simulink model "simulacionrobusto"  (R2024a)
settings: Solver=FixedStepAuto  StartTime=0.0  StopTime=3  FixedStep=0.000001  RelTol=1e-3
model workspace (MAT data in the model file):
  tau = Simulink.Parameter
  tau.Complexity = 'real'
  tau.Dimensions = [0 0]
  tau.DataType = 'auto'
values from neighbouring files (symbols this model uses):
  C = 2610*10^-6    (= 0.00261)    [SITLparameters.m]
  delta1 = 0.022    [SITLparameters.m]
  delta2 = 0.012    [SITLparameters.m]
  E = 12    [SITLparameters.m]
  k1 = 10000    [SITLparameters.m]
  k2 = 280    [SITLparameters.m]
  k3 = 10    [SITLparameters.m]
  kl = 1    [SITLparameters.m]
  kp = 0.0019    [SITLparameters.m]
  kp1 = 0.0019    [SITLparameters.m]
  kp2 = 0.1    [SITLparameters.m]
  kp3 = 0.1    [SITLparameters.m]
  kr1 = 0    [SITLparameters.m]
  kr2 = 0    [SITLparameters.m]
  L = 2010*10^-6    (= 0.00201)    [SITLparameters.m]
  L1 = 0.91    [SITLparameters.m]
  M = 1    [SITLparameters.m]
  R = 25    [SITLparameters.m]
  vd = -8    [SITLparameters.m]
libraries: simulink x6, spsDCVoltageSourceLib x2, spsSawtoothGeneratorLib x2, spsSeriesRLCBranchLib x2, spsCurrentMeasurementLib x1, spsDiodeLib x1, spsMosfetLib x1, slpidlib x1, spsVariableResistorLib x1, spsVoltageMeasurementLib x1, spspowerguiLib x1
settings Model: Creator=LAPONE  LastModifiedBy=rodol
settings SolverCC: ZeroCrossAlgorithm=Adaptive
settings DebuggingCC: IgnoredZcDiagnostic=none  UnconnectedInputMsg=warning  UnconnectedOutputMsg=warning  UnconnectedLineMsg=warning
settings ModelReferenceCC: EnableRefExpFcnMdlSchedulingChecks=on
settings RTWCC: GPUComputeCapability=3.5  DLArmComputeVersion=19.05

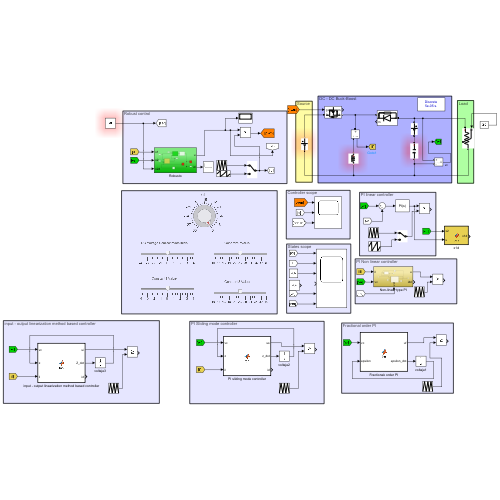
[thumbnail: Simulink's stored preview of the top-level diagram]
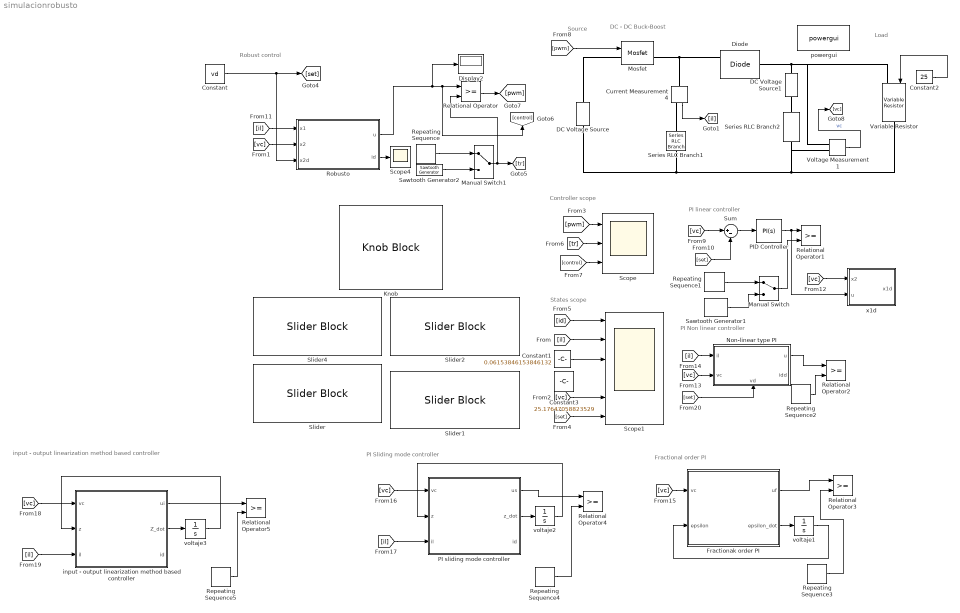
== system simulacionrobusto ==
  note: input - output linearization method based controller
  note: PI Sliding mode controller
  note: Controller scope
  note: States scope
  note: DC - DC Buck-Boost
  note: Robust control
  note: PI linear controller
  note: Load
  note: Source
  note: PI Non linear controller
  note: Fractional order PI
  Constant : Constant  Value=vd
  Constant1 : Constant  Value=0.06153846153846132
  Constant2 : Constant  Value=25
  Constant3 : Constant  Value=25.17647058823529
  Current Measurement4 : spsCurrentMeasurementLib/Current Measurement  PhasorSimulation=off  OutputType=Magnitude  PSBequivalent=0
  DC Voltage Source : spsDCVoltageSourceLib/DC Voltage Source  Amplitude=E  Measurements=Voltage
  DC Voltage Source1 : spsDCVoltageSourceLib/DC Voltage Source  Amplitude=0.06015037593985006  Measurements=None
  Diode : spsDiodeLib/Diode  Ron=0.001  Lon=0  Vf=0.8  IC=0  UseSnubber=0  Rs=500  Cs=250e-9  Measurements=on
  Display2 : Display
  Fractionak order PI : MATLAB Function  TreatAsAtomicUnit=on
  Knob : KnobBlock  ScaleMin=-30  ScaleMax=0
  Manual Switch : ManualSwitch
  Manual Switch1 : ManualSwitch
  Mosfet : spsMosfetLib/Mosfet  Ron=0.1  Lon=0  Rd=0.01  Vfd=0  IC=0  Rs=1e5  Cs=inf  Measurements=on
  Non-linear type PI : Subsystem
      settings: PortSchema="{\"entries\":[{\"content\":{\"sides\":[{\"content\":{\"connectorIds\":[\"In1\",\"In2\"]},\"type\":\"ConnectorPlacement.EquallySpacedRectSide\",\"uuid\":\"ed7c5662-06a7-4150-980f-e3f73a076c84\"},{\"content\":{\"connectorIds\":[\"Out1\",\"Out2\"],\"side\":\"RIGHT\"},\"type\":\"ConnectorPlacement.EquallySpacedRectSide\",\"uuid\":\"55f1d9ea-a8a2-4916-989d-d66eec8a480a\"},{\"content\":{\"connectorIds\":[],\"side\":\"TOP\"},\"type\":\"ConnectorPlacement.EquallySpacedRectSide\",\"uuid\":\"5518ff96-47b6-4e6e-a246-9c294d116829\"},{\"content\":{\"connectorIds\":[\"In3\"],\"side\":\"BOTTOM\"},\"type\":\"ConnectorPlacement.EquallySpacedRectSide\",\"uuid\":\"6100afcc-fe1c-4b13-8923-837ede617b61\"}]},\"type\":\"ConnectorPlacement.EquallySpacedConnector\",\"uuid\":\"24c72a69-ef8d-4d68-8dc5-27cf2fc34569\"}],\"packageUris\":[\"http://schema.mathworks.com/mf0/Connector/R2020b\"],\"version\":\"1.0\"}"
  PI sliding mode controller : MATLAB Function  TreatAsAtomicUnit=on
  PID Controller : slpidlib/PID Controller  Controller=PI  Form=Parallel  TimeDomain=Continuous-time  UseExternalTs=off  SampleTime=-1  IntegratorMethod=Forward Euler  FilterMethod=Forward Euler  ControllerParametersSource=internal  P=0.1  I=1  UseKiTs=off  D=0  UseExternalDerivativeSource=off  N=100  UseFilter=on  TunerSelectOption=Transfer Function Based (PID Tuner App)  InitialConditionSource=internal  InitialConditionForIntegrator=0  InitialConditionForFilter=0  DifferentiatorICPrevScaledInput=0  ExternalReset=none  TrackingMode=off  Kt=1  LimitOutput=off  SatLimitsSource=internal  UpperSaturationLimit=inf  LowerSaturationLimit=-inf  LinearizeAsGain=on  AntiWindupMode=none  Kb=1  LimitIntegrator=off  UpperIntegratorSaturationLimit=inf  LowerIntegratorSaturationLimit=-inf  POutMin=[]  POutMax=[]  IOutMin=[]  IOutMax=[]  DOutMin=[]  DOutMax=[]  NOutMin=[]  NOutMax=[]  SumOutMin=[]  SumOutMax=[]  SaturationOutMin=[]  SaturationOutMax=[]  PParamMin=[]  PParamMax=[]  IParamMin=[]  IParamMax=[]  DParamMin=[]  DParamMax=[]  NParamMin=[]  NParamMax=[]  KbParamMin=[]  KbParamMax=[]  KtParamMin=[]  KtParamMax=[]  KbOutMin=[]  KbOutMax=[]  KtOutMin=[]  KtOutMax=[]  IntegratorOutMin=[]  IntegratorOutMax=[]  FilterOutMin=[]  FilterOutMax=[]  SumI1OutMin=[]  SumI1OutMax=[]  SumI2OutMin=[]  SumI2OutMax=[]  SumI3OutMin=[]  SumI3OutMax=[]  SumI4OutMin=[]  SumI4OutMax=[]  SumDOutMin=[]  SumDOutMax=[]  DifferentiatorOutMin=[]  DifferentiatorOutMax=[]  FilterDiffOutCoefMin=[]  FilterDiffOutCoefMax=[]  ReciprocalOutMin=[]  ReciprocalOutMax=[]  SumDenOutMin=[]  SumDenOutMax=[]  SumNumOutMin=[]  SumNumOutMax=[]  DivideOutMin=[]  DivideOutMax=[]  UdiffTsProdOutMin=[]  UdiffTsProdOutMax=[]  NTsProdOutMin=[]  NTsProdOutMax=[]  UintegralTsProdOutMin=[]  UintegralTsProdOutMax=[]  UngainTsProdOutMin=[]  UngainTsProdOutMax=[]  ClampingZeroOutDataTypeStr=Inherit: Inherit via back propagation  ClampingZeroOutMin=[]  ClampingZeroOutMax=[]  FilterDenConstantOutDataTypeStr=Inherit: Inherit via back propagation  FilterDenConstantOutMin=[]  FilterDenConstantOutMax=[]  PCopyOutDataTypeStr=Inherit: Inherit via back propagation  PCopyOutMin=[]  PCopyOutMax=[]  NCopyOutDataTypeStr=Inherit: Inherit via back propagation  NCopyOutMin=[]  NCopyOutMax=[]  IntegratorContinuousStateAttributes=''  IntegratorStateMustResolveToSignalObject=off  IntegratorRTWStateStorageClass=Auto  FilterContinuousStateAttributes=''  FilterStateMustResolveToSignalObject=off  FilterRTWStateStorageClass=Auto  ParallelPVariant=InternalParameters  IdealPVariant=Disabled  IVariant=InternalParameters  DVariant=Disabled  IntegratorVariant=Continuous  SatVariant=Disabled  AWVariant=Passthrough  PCopyVariant=Disabled  TRVariant=Disabled  FdbkBlocksVariant=Forward  IdealPFdbkVariant=Disabled  SatFdbkVariant=Disabled  DerivativeFilterVariant=Disabled  NVariant=Disabled  NCopyVariant=Disabled_SignalSpec  FilterICVariant=Disabled  IntegratorICVariant=InternalICs  ExternalResetVariant=Disabled  TRSumVariant=Passthrough  SumFdbkVariant=Disabled  SumVariant=Sum_PI  TsampFilterVariant=InternalTs  TsampNgainVariant=Passthrough  TsampIntegralVariant=Disabled_SignalSpec  ExternalSaturationOutDataTypeStr=Inherit: Same as second input  DerivativeSourceVariant=Disabled
  Relational Operator{,1..5} (6 alike) : RelationalOperator  OutDataTypeStr=boolean  RndMeth=Simplest  InputSameDT=off
  Repeating Sequence{,1..5} (6 alike) : simulink/Sources/Repeating Sequence  rep_seq_t=[0 0.0001 0.0002]  rep_seq_y=[0 1 0]
  Robusto : Subsystem
  Sawtooth Generator1 : spsSawtoothGeneratorLib/Sawtooth Generator  Freq=2000  Phase=180  Ts=0
  Sawtooth Generator2 : spsSawtoothGeneratorLib/Sawtooth Generator  Freq=2000  Phase=180  Ts=0
  Scope : Scope  NumInputPorts=3
  Scope1 : Scope  NumInputPorts=6
  Scope4 : Scope
  Series RLC Branch1 : spsSeriesRLCBranchLib/Series RLC Branch  LConnTagsString=__new0  RConnTagsString=__new0  BranchType=L  Resistance=1  Inductance=L  SetiL0=off  InitialCurrent=0  Capacitance=1e-6  Setx0=off  InitialVoltage=0  Measurements=None
  Series RLC Branch2 : spsSeriesRLCBranchLib/Series RLC Branch  LConnTagsString=__new0  RConnTagsString=__new0  BranchType=C  Resistance=1  Inductance=1e-3  SetiL0=off  InitialCurrent=0  Capacitance=C  Setx0=off  InitialVoltage=0  Measurements=None
  Slider : SliderBlock  ScaleMin=-4  ScaleMax=4
  Slider1 : SliderBlock  ScaleMin=10  ScaleMax=40
  Slider2 : SliderBlock  ScaleMin=10  ScaleMax=40
  Slider4 : SliderBlock  ScaleMin=-4  ScaleMax=4
  Sum : Sum  Inputs=|+-
  Variable Resistor : spsVariableResistorLib/Variable Resistor  Rabsmin=1e-3
  Voltage Measurement1 : spsVoltageMeasurementLib/Voltage Measurement  PhasorSimulation=off  OutputType=Complex  PSBequivalent=0
  input - output linearization method based controller : MATLAB Function  TreatAsAtomicUnit=on
  powergui : spspowerguiLib/powergui  Priority=1  SimulationMode=Discrete  SampleTime=50e-6  frequency=60  Iterations=50  frequencyindice=0  Pbase=100e6  ErrMax=1e-4  UnitsV=kV  UnitsW=MW  buscounter=0  FunctionMessages=off  echomessages=off  EnableUseOfTLC=off  CurrentSourceSwitches=off  DisableSnubberDevices=off  DisableRonSwitches=off  DisableVfSwitches=off  DisplayEquations=off  AutomaticDiscreteSolvers=off  SolverType=Tustin/Backward Euler (TBE)  Interpol=off  ExternalGateDelay=off  methode=off  Ts=100  x0status=blocks  SPID=on  SwTol=0  HookPort=off  NonlinearTolerance=1e-4  nMaxIteration=100  ContinueOnMaxIteration=off  RestoreLinks=warning  ResistiveCurrentMeasurement=off  Frange=[0:2:500]  Ylog=off  Xlog=on  ShowGrid=off  save=off  variable=ZData  structure=0  ZoomFFT=off  StartTime=0.0  cycles=1  DisplayStyle=1  fundamental=60  FreqAxis=off  MaxFrequency=1000  frequencyindicesteady=1  RmsSteady=1  display=off
  voltaje1 : Integrator
  voltaje2 : Integrator
  voltaje3 : Integrator
  x1d : MATLAB Function  TreatAsAtomicUnit=on
  wires:
  [il] -> Scope1/2
  [id] -> Scope1/1
  Voltage Measurement1/1 -> [vc]  "vc"
  Sum/1 -> PID Controller/1
  [set] -> Scope1/6
  [set] -> Sum/2
  [pwm] -> Mosfet/1
  Manual Switch/1 -> Relational Operator1/2
  [vc] -> Sum/1
  Sawtooth Generator2/1 -> Manual Switch1/2
  [vc] -> x1d/1(x2)
  Repeating Sequence1/1 -> Manual Switch/1
  [vc] -> Robusto/2(x2)
  Constant1/1 -> Scope1/3
  [tr] -> Scope/2
  [vc] -> Scope1/5
  Sawtooth Generator1/1 -> Manual Switch/2
  [control] -> Scope/3
  PID Controller/1 -> x1d/2(u), Relational Operator1/1
  Repeating Sequence/1 -> Manual Switch1/1
  [pwm] -> Scope/1
  [vc] -> Non-linear type PI/2(vc)
  [il] -> Non-linear type PI/1(il)
  Repeating Sequence2/1 -> Relational Operator2/2
  Fractionak order PI/1(uf) -> Relational Operator3/1
  Repeating Sequence3/1 -> Relational Operator3/2
  Fractionak order PI/2(epsilon_dot) -> voltaje1/1
  voltaje1/1 -> Fractionak order PI/2(epsilon)
  [vc] -> Fractionak order PI/1(vc)
  PI sliding mode controller/2(z_dot) -> voltaje2/1
  voltaje2/1 -> PI sliding mode controller/2(z)
  [vc] -> PI sliding mode controller/1(vc)
  [il] -> PI sliding mode controller/3(il)
  PI sliding mode controller/1(us) -> Relational Operator4/1
  Repeating Sequence4/1 -> Relational Operator4/2
  input - output linearization method based controller/2(Z_dot) -> voltaje3/1
  voltaje3/1 -> input - output linearization method based controller/2(z)
  input - output linearization method based controller/1(ui) -> Relational Operator5/1
  Repeating Sequence5/1 -> Relational Operator5/2
  [vc] -> input - output linearization method based controller/1(vc)
  [il] -> input - output linearization method based controller/3(il)
  [il] -> Robusto/1(x1)
  Non-linear type PI/1(u) -> Relational Operator2/1
  [set] -> Non-linear type PI/3(vd)
  Constant/1 -> Robusto/3(x2d), [set]
  Constant2/1 -> Variable Resistor/1
  Manual Switch1/1 -> [tr], Relational Operator/2
  Relational Operator/1 -> [pwm]
  Robusto/2(id) -> Scope4/1
  Robusto/1(u) -> [control], Relational Operator/1, Display2/1
  Current Measurement4/1 -> [il]
  connections:
  DC Voltage Source1/RConn1 -- Voltage Measurement1/LConn1 -- Variable Resistor/LConn1 -- Diode/LConn1
  Variable Resistor/RConn1 -- Voltage Measurement1/LConn2 -- Series RLC Branch2/RConn1 -- Series RLC Branch1/RConn1 -- DC Voltage Source/LConn1
  DC Voltage Source1/LConn1 -- Series RLC Branch2/LConn1
  Mosfet/RConn1 -- Diode/RConn1 -- Current Measurement4/LConn1
  Mosfet/LConn1 -- DC Voltage Source/RConn1
  Current Measurement4/RConn1 -- Series RLC Branch1/LConn1

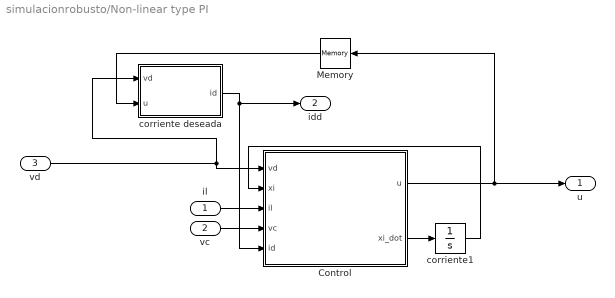
== system simulacionrobusto/Non-linear type PI ==
  il : Inport
  vc : Inport  Port=2
  vd : Inport  Port=3
  Control : MATLAB Function  TreatAsAtomicUnit=on
  Memory : Memory
  corriente deseada : MATLAB Function  TreatAsAtomicUnit=on
  corriente1 : Integrator  InitialCondition=0.001
  u : Outport
  idd : Outport  Port=2
  wires:
  Control/2(xi_dot) -> corriente1/1
  corriente1/1 -> Control/2(xi)
  Control/1(u) -> Memory/1, u/1
  vd/1 -> corriente deseada/1(vd), Control/1(vd)
  il/1 -> Control/3(il)
  vc/1 -> Control/4(vc)
  Memory/1 -> corriente deseada/2(u)
  corriente deseada/1(id) -> idd/1, Control/5(id)

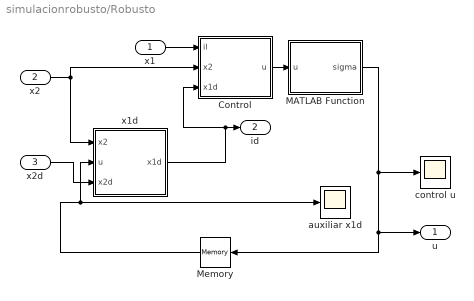
== system simulacionrobusto/Robusto ==
  x1 : Inport
  x2 : Inport  Port=2
  x2d : Inport  Port=3
  Control : MATLAB Function  TreatAsAtomicUnit=on
  MATLAB Function : MATLAB Function  TreatAsAtomicUnit=on
  Memory : Memory
  auxiliar x1d : Scope
  control u : Scope
  x1d : MATLAB Function  TreatAsAtomicUnit=on
  u : Outport
  id : Outport  Port=2
  wires:
  x1/1 -> Control/1(il)
  x2/1 -> x1d/1(x2), Control/2(x2)
  Memory/1 -> x1d/2(u), auxiliar x1d/1
  x2d/1 -> x1d/3(x2d)
  x1d/1(x1d) -> Control/3(x1d), id/1
  MATLAB Function/1(sigma) -> Memory/1, u/1, control u/1
  Control/1(u) -> MATLAB Function/1(u)

== matlab function simulacionrobusto/input - output linearization method based controller ==
  data: kp3 parameter; vc input; ui output; Z_dot output; kl parameter; z input; il input; vd parameter; k3 parameter; E parameter; id output
function [ui,Z_dot,id] = fcn(kp3,vc,kl,z, il,vd,k3,E)

ev = vc - vd ;
Z_dot = ev;
id = kp3*ev + k3*z;

ui = (-vc - kl*(il - id))/ (E - vc);

== matlab function simulacionrobusto/Robusto/MATLAB Function ==
  data: u input; sigma output; L1 parameter; M parameter
function sigma  = fcn(u, L1, M)
    amin = (pi) / (2 * (M - L1));
    s = u;
    if s < L1
        sigma = s;
    elseif s >= L1
        %sigma = tanh(amin * (s - L1)) / amin + L1;
        sigma = (1 / amin) * tanh(amin * (s - L1)) + L1;
    else
        sigma = 0;
    end
end

== matlab function simulacionrobusto/Robusto/Control ==
  data: il input; u output; x2 input; x1d input; E parameter; L parameter; kr1 parameter
function u = control(il, x2, x1d, E, L, kr1)

%error
e1 = il - x1d;

%control
%u = ( E + kr1*L*sign(e1) ) / ( x2 - E) + 1;
u = L * (kr1 * sqrt(abs(e1)) * sign(e1) + E / L) / (x2 - E) + 1;
%u = L * (kr1 * (e1) + E / L) / (x2 - E) + 1;
end

== matlab function simulacionrobusto/x1d ==
  data: x1d output; x2 input; u input; C parameter; R parameter; k2 parameter; vd parameter
function x1d = des(x2, u, C, R, k2, vd)

%error
e2 = x2 - vd;

%Auxiliar control
x1d = ( k2*C*sign(e2) - x2/R ) / (1-u);

== matlab function simulacionrobusto/Robusto/x1d ==
  data: x1d output; x2 input; u input; C parameter; R parameter; x2d input; kr2 parameter
function x1d = des(x2, u, C, R,x2d, kr2)

%error
e2 = x2 - x2d;

%Auxiliar control
x1d = C * (kr2 * sqrt(abs(e2)) * sign(e2) - (1 / (R * C)) * (e2 + x2d)) / (1 - u);

== matlab function simulacionrobusto/Non-linear type PI/Control ==
  data: E parameter; R parameter; kp parameter; vd input; xi input; il input; u output; vc input; xi_dot output; L parameter; delta2 parameter; delta1 parameter; id input
function [u,xi_dot] = fcn(E, R, kp, vd, xi,il,vc,L, delta2, delta1, id)

ei_s = il - id - xi ;    ev = vc - vd ;

gamma  = (delta1 - delta2)/(L*delta1*delta2);
phi = -kp*((delta1*(E - vd)*ei_s) + delta2*vd*((vd-E)/R*E)*ev );
xi_dot = -gamma*delta2*((E/(vd - E)+ phi)*ev);
u = (vd/(vd-E))+ phi;

== matlab function simulacionrobusto/Non-linear type PI/corriente deseada ==
  data: vd input; R parameter; id output; u input
function id  = fcn(vd,R,u)

id = (vd/(R*(1-u)));

== matlab function simulacionrobusto/Fractionak order PI ==
  data: kp1 parameter; vc input; k1 parameter; uf output; epsilon_dot output; epsilon input; vd parameter
function [uf,epsilon_dot] = fcn(kp1,vc,k1,epsilon, vd)

ev = vc - vd ;

epsilon_dot = ev;
uf = kp1*ev + k1+epsilon;

== matlab function simulacionrobusto/PI sliding mode controller ==
  data: kp2 parameter; vc input; us output; z_dot output; k2 parameter; z input; il input; vd parameter; id output
function [us,z_dot,id] = fcn(kp2,vc,k2,z, il,vd)

ev = vc - vd ;
z_dot = ev;
id = kp2*ev + k2*z;

us = (1/2)*(1 - sign(il - id));
